simulink model "solar_PV_model"  (R2019a)
settings: Solver=VariableStepAuto  StartTime=0.0  StopTime=80  RelTol=1e-3
undefined symbols (not defined in the file or in its folder): BM, Eg0, Isc, J, K, Kc, ki, La, n, Ns, q, Ra, Rs, Rsh, Tn, Voc
libraries: simulink_extras x4, simulink x2
settings Model: Creator=hermi  LastModifiedBy=hermi

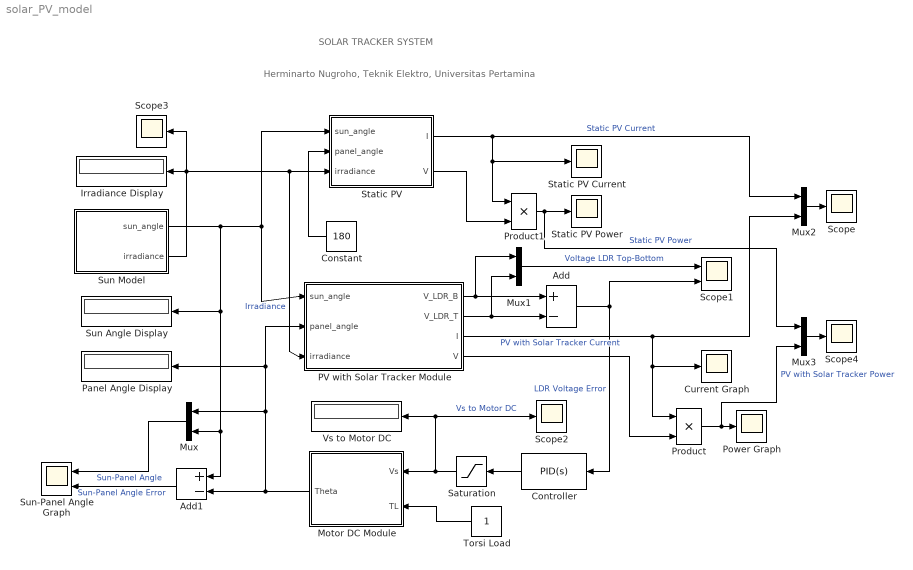
== system solar_PV_model ==
  note: Herminarto Nugroho, Teknik Elektro, Universitas Pertamina
  note: SOLAR TRACKER SYSTEM
  Add : Sum  Inputs=+-
  Add1 : Sum  Inputs=+-
  Constant : Constant  Value=180
  Controller : simulink/Continuous/PID Controller  Controller=PID  Form=Parallel  TimeDomain=Continuous-time  SampleTime=-1  IntegratorMethod=Forward Euler  FilterMethod=Forward Euler  ControllerParametersSource=internal  P=100  I=100  D=0  UseFilter=on  N=100  TunerSelectOption=Transfer Function Based (PID Tuner App)  InitialConditionSource=internal  InitialConditionForIntegrator=0  InitialConditionForFilter=0  DifferentiatorICPrevScaledInput=0  ExternalReset=none  TrackingMode=off  Kt=1  LimitOutput=off  UpperSaturationLimit=180  LowerSaturationLimit=0  LinearizeAsGain=on  AntiWindupMode=none  Kb=1  POutMin=[]  POutMax=[]  IOutMin=[]  IOutMax=[]  DOutMin=[]  DOutMax=[]  NOutMin=[]  NOutMax=[]  SumOutMin=[]  SumOutMax=[]  SaturationOutMin=[]  SaturationOutMax=[]  PParamMin=[]  PParamMax=[]  IParamMin=[]  IParamMax=[]  DParamMin=[]  DParamMax=[]  NParamMin=[]  NParamMax=[]  KbParamMin=[]  KbParamMax=[]  KtParamMin=[]  KtParamMax=[]  KbOutMin=[]  KbOutMax=[]  KtOutMin=[]  KtOutMax=[]  IntegratorOutMin=[]  IntegratorOutMax=[]  FilterOutMin=[]  FilterOutMax=[]  SumI1OutMin=[]  SumI1OutMax=[]  SumI2OutMin=[]  SumI2OutMax=[]  SumI3OutMin=[]  SumI3OutMax=[]  SumI4OutMin=[]  SumI4OutMax=[]  SumDOutMin=[]  SumDOutMax=[]  DifferentiatorOutMin=[]  DifferentiatorOutMax=[]  FilterDiffOutCoefMin=[]  FilterDiffOutCoefMax=[]  ReciprocalOutMin=[]  ReciprocalOutMax=[]  SumDenOutMin=[]  SumDenOutMax=[]  SumNumOutMin=[]  SumNumOutMax=[]  DivideOutMin=[]  DivideOutMax=[]  IntegratorContinuousStateAttributes=''  IntegratorStateMustResolveToSignalObject=off  IntegratorRTWStateStorageClass=Auto  FilterContinuousStateAttributes=''  FilterStateMustResolveToSignalObject=off  FilterRTWStateStorageClass=Auto  ParallelPVariant=InternalParameters  IdealPVariant=Disabled  IVariant=InternalParameters  DVariant=InternalParameters  IntegratorVariant=Continuous  SatVariant=Disabled  AWVariant=Passthrough  PCopyVariant=Disabled  TRVariant=Disabled  FdbkBlocksVariant=Forward  IdealPFdbkVariant=Disabled  SatFdbkVariant=Disabled  DerivativeFilterVariant=ContFilter  NVariant=InternalParameters  NCopyVariant=Disabled  FilterICVariant=InternalICsFilter  IntegratorICVariant=InternalICs  ExternalResetVariant=Disabled  TRSumVariant=Passthrough  SumFdbkVariant=Disabled  SumVariant=Sum_PID
  Current Graph : Scope
  Irradiance Display : Display
  Motor DC Module : Subsystem  InitFcn=|
      | Ra=0.5,
      | La=1.5e-3,
      | Kc=0.05,
      | J=2.5e-4,
      | BM=1e-4,
  Mux{,1..3} (4 alike) : Mux  Inputs=2
  PV with Solar Tracker Module : Subsystem
  Panel Angle Display : Display
  Power Graph : Scope
  Product : Product
  Product1 : Product
  Saturation : Saturate  UpperLimit=12  LowerLimit=-12
  Scope{,2..4} (4 alike) : Scope
  Scope1 : Scope  NumInputPorts=2
  Static PV : Subsystem
  Static PV Current : Scope
  Static PV Power : Scope
  Sun Angle Display : Display
  Sun Model : Subsystem
  Sun-Panel Angle Graph : Scope  NumInputPorts=2
  Torsi Load : Constant
  Vs to Motor DC : Display
  wires:
  PV with Solar Tracker Module/3(I) -> Mux2/2, Current Graph/1, Product/1  "PV with Solar Tracker Current"
  PV with Solar Tracker Module/4(V) -> Product/2
  Product/1 -> Mux3/2, Power Graph/1  "PV with Solar Tracker Power"
  Sun Model/2(irradiance) -> PV with Solar Tracker Module/3(irradiance), Static PV/3(irradiance), Scope3/1, Irradiance Display/1  "Irradiance"
  Motor DC Module/1(Theta) -> Add1/2, Mux/1, Panel Angle Display/1, PV with Solar Tracker Module/2(panel_angle)
  Add/1 -> Scope1/2, Controller/1  "LDR Voltage Error"
  Sun Model/1(sun_angle) -> Add1/1, Mux/2, Sun Angle Display/1, Static PV/1(sun_angle), PV with Solar Tracker Module/1(sun_angle)
  PV with Solar Tracker Module/1(V_LDR_B) -> Mux1/1, Add/1
  PV with Solar Tracker Module/2(V_LDR_T) -> Mux1/2, Add/2
  Torsi Load/1 -> Motor DC Module/2(TL)
  Controller/1 -> Saturation/1
  Saturation/1 -> Scope2/1, Vs to Motor DC/1, Motor DC Module/1(Vs)  "Vs to Motor DC"
  Mux/1 -> Sun-Panel Angle Graph/1  "Sun-Panel Angle"
  Add1/1 -> Sun-Panel Angle Graph/2  "Sun-Panel Angle Error"
  Mux1/1 -> Scope1/1  "Voltage LDR Top-Bottom"
  Product1/1 -> Static PV Power/1, Mux3/1  "Static PV Power"
  Static PV/1(I) -> Product1/1, Static PV Current/1, Mux2/1  "Static PV Current"
  Static PV/2(V) -> Product1/2
  Mux2/1 -> Scope/1
  Constant/1 -> Static PV/2(panel_angle)
  Mux3/1 -> Scope4/1

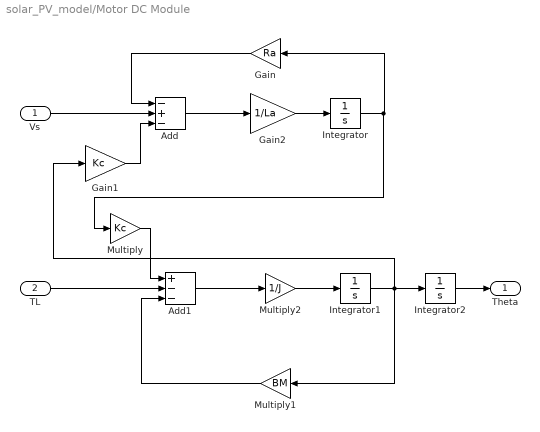
== system solar_PV_model/Motor DC Module ==
  Vs : Inport
  TL : Inport  Port=2
  Add : Sum  Inputs=-+-
  Add1 : Sum  Inputs=+--
  Gain : Gain  Gain=Ra
  Gain1 : Gain  Gain=Kc
  Gain2 : Gain  Gain=1/La
  Integrator : Integrator
  Integrator1 : Integrator
  Integrator2 : Integrator
  Multiply : Gain  Gain=Kc
  Multiply1 : Gain  Gain=BM
  Multiply2 : Gain  Gain=1/J
  Theta : Outport
  wires:
  Gain1/1 -> Add/3
  Gain/1 -> Add/1
  Multiply/1 -> Add1/1
  Add1/1 -> Multiply2/1
  Gain2/1 -> Integrator/1
  TL/1 -> Add1/2
  Multiply2/1 -> Integrator1/1
  Integrator1/1 -> Integrator2/1, Multiply1/1, Gain1/1
  Add/1 -> Gain2/1
  Vs/1 -> Add/2
  Integrator/1 -> Multiply/1, Gain/1
  Multiply1/1 -> Add1/3
  Integrator2/1 -> Theta/1

== system solar_PV_model/PV with Solar Tracker Module ==
  sun_angle : Inport
  panel_angle : Inport  Port=2
  irradiance : Inport  Port=3
  Effective Irradiance Model : Subsystem
  LDR Sensor Module : Subsystem
  PV Module : Subsystem  InitFcn=|
      | ki=0.0032,
      | q=1.6e-19,
      | K=1.38e-23,
      | n=1.3,
      | Eg0=1.1,
      | Rs=0.221,
      | Rsh=414.405,
      | Tn=298,
      | Voc=32.9,
      | Isc=8.21,
      | Ns=54,
  Temperature (C) : Constant  Value=30
  V_LDR_B : Outport
  V_LDR_T : Outport  Port=2
  I : Outport  Port=3
  V : Outport  Port=4
  wires:
  sun_angle/1 -> Effective Irradiance Model/1(sun_angle), LDR Sensor Module/1(sun_angle)
  panel_angle/1 -> Effective Irradiance Model/2(panel_angle), LDR Sensor Module/2(panel_angle)
  Temperature (C)/1 -> PV Module/1(T)
  Effective Irradiance Model/1(effective_irradiance) -> PV Module/2(G)
  LDR Sensor Module/1(V_LDR_B1) -> V_LDR_B/1
  irradiance/1 -> Effective Irradiance Model/3(irradiance), LDR Sensor Module/3(irradiance)
  LDR Sensor Module/2(V_LDR_T1) -> V_LDR_T/1
  PV Module/1(I) -> I/1  "PV Current"
  PV Module/2(V) -> V/1  "V"

== system solar_PV_model/Static PV ==
  sun_angle : Inport
  panel_angle : Inport  Port=2
  irradiance : Inport  Port=3
  Effective Irradiance Model : Subsystem
  PV Module : Subsystem  InitFcn=|
      | ki=0.0032,
      | q=1.6e-19,
      | K=1.38e-23,
      | n=1.3,
      | Eg0=1.1,
      | Rs=0.221,
      | Rsh=414.405,
      | Tn=298,
      | Voc=32.9,
      | Isc=8.21,
      | Ns=54,
  Temperature (C) : Constant  Value=30
  I : Outport
  V : Outport  Port=2
  wires:
  Temperature (C)/1 -> PV Module/1(T)
  Effective Irradiance Model/1(effective_irradiance) -> PV Module/2(G)
  sun_angle/1 -> Effective Irradiance Model/1(sun_angle)
  panel_angle/1 -> Effective Irradiance Model/2(panel_angle)
  irradiance/1 -> Effective Irradiance Model/3(irradiance)
  PV Module/1(I) -> I/1  "PV Current"
  PV Module/2(V) -> V/1  "V"

== system solar_PV_model/Sun Model ==
  15_deg/hr : Constant  Value=15/60
  MATLAB Function : MATLAB Function  TreatAsAtomicUnit=on
  Product1 : Product
  Saturation : Saturate  UpperLimit=18*60  LowerLimit=6*60
  Starting 6 am : simulink/Sources/Ramp  slope=10  start=0  InitialOutput=6*60
  sun_angle : Outport
  irradiance : Outport  Port=2
  wires:
  15_deg/hr/1 -> Product1/2
  Starting 6 am/1 -> Saturation/1
  MATLAB Function/1(X) -> irradiance/1
  Saturation/1 -> MATLAB Function/1(x), Product1/1
  Product1/1 -> sun_angle/1

== system solar_PV_model/PV with Solar Tracker Module/Effective Irradiance Model ==
  sun_angle : Inport
  panel_angle : Inport  Port=2
  irradiance : Inport  Port=3
  Add : Sum  Inputs=+-
  Cos : Trigonometry  Operator=cos
  Degrees to Radians : simulink_extras/Transformations/Degrees to Radians
  Product2 : Product  Inputs=**
  Saturation : Saturate  UpperLimit=90  LowerLimit=-90
  effective_irradiance : Outport
  wires:
  sun_angle/1 -> Add/1
  Cos/1 -> Product2/1
  Product2/1 -> effective_irradiance/1
  Degrees to Radians/1 -> Cos/1
  Add/1 -> Degrees to Radians/1
  panel_angle/1 -> Add/2
  irradiance/1 -> Product2/2

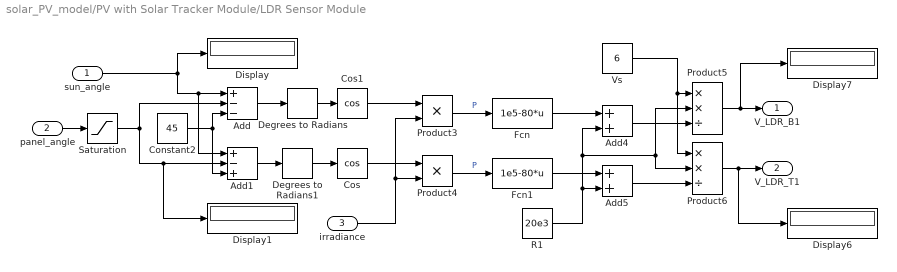
== system solar_PV_model/PV with Solar Tracker Module/LDR Sensor Module ==
  sun_angle : Inport
  panel_angle : Inport  Port=2
  irradiance : Inport  Port=3
  Add : Sum  Inputs=+--
  Add1 : Sum  Inputs=+-+
  Add4 : Sum
  Add5 : Sum
  Constant2 : Constant  Value=45
  Cos : Trigonometry  Operator=cos
  Cos1 : Trigonometry  Operator=cos
  Degrees to Radians : simulink_extras/Transformations/Degrees to Radians
  Degrees to Radians1 : simulink_extras/Transformations/Degrees to Radians
  Display{,1,6..7} (4 alike) : Display
  Fcn : Fcn  Expr=1e5-80*u
  Fcn1 : Fcn  Expr=1e5-80*u
  Product3 : Product
  Product4 : Product
  Product5 : Product  Inputs=**/
  Product6 : Product  Inputs=**/
  R1 : Constant  Value=20e3
  Saturation : Saturate  UpperLimit=360  LowerLimit=0
  Vs : Constant  Value=6
  V_LDR_B1 : Outport
  V_LDR_T1 : Outport  Port=2
  wires:
  Product6/1 -> Display6/1, V_LDR_T1/1
  Add4/1 -> Product5/3
  Vs/1 -> Product6/1, Product5/1
  R1/1 -> Add5/2, Product6/2, Product5/2, Add4/2
  irradiance/1 -> Product4/2, Product3/2
  Degrees to Radians1/1 -> Cos/1
  Add5/1 -> Product6/3
  Product5/1 -> Display7/1, V_LDR_B1/1
  Add1/1 -> Degrees to Radians1/1
  Cos1/1 -> Product3/1
  Product4/1 -> Fcn1/1  "P"
  Cos/1 -> Product4/1
  Fcn/1 -> Add4/1
  Product3/1 -> Fcn/1  "P"
  Add/1 -> Degrees to Radians/1
  Constant2/1 -> Add1/3, Add/3
  Degrees to Radians/1 -> Cos1/1
  panel_angle/1 -> Saturation/1
  sun_angle/1 -> Add1/1, Add/1, Display/1
  Fcn1/1 -> Add5/1
  Saturation/1 -> Add/2, Display1/1, Add1/2

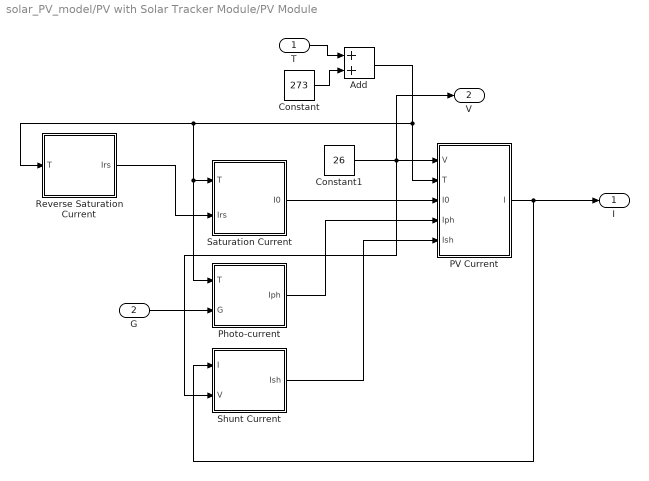
== system solar_PV_model/PV with Solar Tracker Module/PV Module ==
  T : Inport
  G : Inport  Port=2
  Add : Sum
  Constant : Constant  Value=273
  Constant1 : Constant  Value=26
  PV Current : Subsystem
  Photo-current : Subsystem
  Reverse Saturation Current : Subsystem
  Saturation Current : Subsystem
  Shunt Current : Subsystem
  I : Outport
  V : Outport  Port=2
  wires:
  Photo-current/1(Iph) -> PV Current/4(Iph)
  Saturation Current/1(I0) -> PV Current/3(I0)
  PV Current/1(I) -> I/1, Shunt Current/1(I)
  G/1 -> Photo-current/2(G)
  Add/1 -> PV Current/2(T), Reverse Saturation Current/1(T), Saturation Current/1(T), Photo-current/1(T)
  Constant/1 -> Add/2
  Constant1/1 -> V/1, Shunt Current/2(V), PV Current/1(V)
  Shunt Current/1(Ish) -> PV Current/5(Ish)
  Reverse Saturation Current/1(Irs) -> Saturation Current/2(Irs)
  T/1 -> Add/1

== system solar_PV_model/Static PV/Effective Irradiance Model ==
  sun_angle : Inport
  panel_angle : Inport  Port=2
  irradiance : Inport  Port=3
  Add : Sum  Inputs=+-
  Cos : Trigonometry  Operator=cos
  Degrees to Radians : simulink_extras/Transformations/Degrees to Radians
  Product2 : Product  Inputs=**
  Saturation : Saturate  UpperLimit=90  LowerLimit=-90
  effective_irradiance : Outport
  wires:
  sun_angle/1 -> Add/1
  Cos/1 -> Product2/1
  Product2/1 -> effective_irradiance/1
  Degrees to Radians/1 -> Cos/1
  Add/1 -> Degrees to Radians/1
  panel_angle/1 -> Add/2
  irradiance/1 -> Product2/2

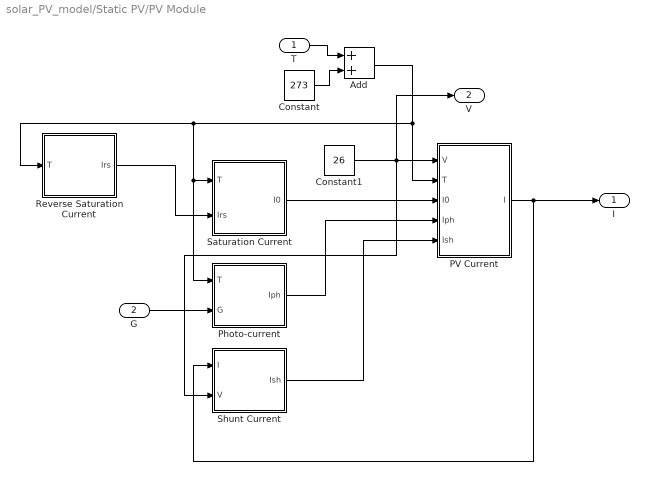
== system solar_PV_model/Static PV/PV Module ==
  T : Inport
  G : Inport  Port=2
  Add : Sum
  Constant : Constant  Value=273
  Constant1 : Constant  Value=26
  PV Current : Subsystem
  Photo-current : Subsystem
  Reverse Saturation Current : Subsystem
  Saturation Current : Subsystem
  Shunt Current : Subsystem
  I : Outport
  V : Outport  Port=2
  wires:
  Photo-current/1(Iph) -> PV Current/4(Iph)
  Saturation Current/1(I0) -> PV Current/3(I0)
  PV Current/1(I) -> I/1, Shunt Current/1(I)
  G/1 -> Photo-current/2(G)
  Add/1 -> PV Current/2(T), Reverse Saturation Current/1(T), Saturation Current/1(T), Photo-current/1(T)
  Constant/1 -> Add/2
  Constant1/1 -> V/1, Shunt Current/2(V), PV Current/1(V)
  Shunt Current/1(Ish) -> PV Current/5(Ish)
  Reverse Saturation Current/1(Irs) -> Saturation Current/2(Irs)
  T/1 -> Add/1

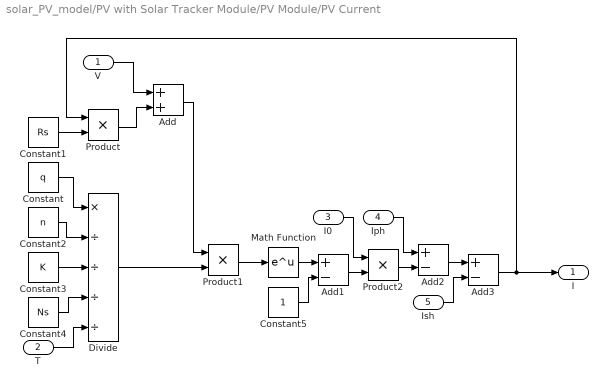
== system solar_PV_model/PV with Solar Tracker Module/PV Module/PV Current ==
  V : Inport
  T : Inport  Port=2
  I0 : Inport  Port=3
  Iph : Inport  Port=4
  Ish : Inport  Port=5
  Add : Sum
  Add1 : Sum  Inputs=+-
  Add2 : Sum  Inputs=+-
  Add3 : Sum  Inputs=+-
  Constant : Constant  Value=q
  Constant1 : Constant  Value=Rs
  Constant2 : Constant  Value=n
  Constant3 : Constant  Value=K
  Constant4 : Constant  Value=Ns
  Constant5 : Constant
  Divide : Product  Inputs=*////
  Math Function : Math  SaturateOnIntegerOverflow=on
  Product : Product
  Product1 : Product
  Product2 : Product
  I : Outport
  wires:
  Constant5/1 -> Add1/2
  Add1/1 -> Product2/2
  Constant3/1 -> Divide/3
  Add/1 -> Product1/1
  T/1 -> Divide/5
  Divide/1 -> Product1/2
  Constant2/1 -> Divide/2
  Product1/1 -> Math Function/1
  Product2/1 -> Add2/2
  Iph/1 -> Add2/1
  Math Function/1 -> Add1/1
  Constant1/1 -> Product/2
  Product/1 -> Add/2
  V/1 -> Add/1
  I0/1 -> Product2/1
  Constant/1 -> Divide/1
  Add2/1 -> Add3/1
  Add3/1 -> I/1, Product/1
  Constant4/1 -> Divide/4
  Ish/1 -> Add3/2

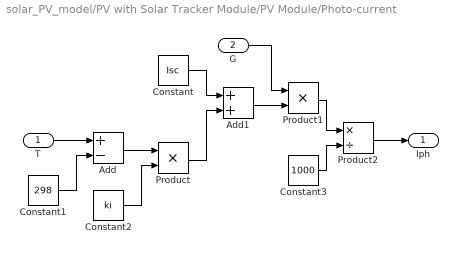
== system solar_PV_model/PV with Solar Tracker Module/PV Module/Photo-current ==
  T : Inport
  G : Inport  Port=2
  Add : Sum  Inputs=+-
  Add1 : Sum
  Constant : Constant  Value=Isc
  Constant1 : Constant  Value=298
  Constant2 : Constant  Value=ki
  Constant3 : Constant  Value=1000
  Product : Product
  Product1 : Product
  Product2 : Product  Inputs=*/
  Iph : Outport
  wires:
  T/1 -> Add/1
  Add/1 -> Product/1
  Constant/1 -> Add1/1
  Product1/1 -> Product2/1
  Product2/1 -> Iph/1
  G/1 -> Product1/1
  Add1/1 -> Product1/2
  Constant3/1 -> Product2/2
  Constant1/1 -> Add/2
  Constant2/1 -> Product/2
  Product/1 -> Add1/2

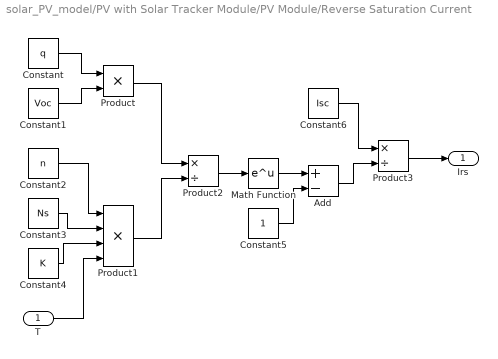
== system solar_PV_model/PV with Solar Tracker Module/PV Module/Reverse Saturation Current ==
  T : Inport
  Add : Sum  Inputs=+-
  Constant : Constant  Value=q
  Constant1 : Constant  Value=Voc
  Constant2 : Constant  Value=n
  Constant3 : Constant  Value=Ns
  Constant4 : Constant  Value=K
  Constant5 : Constant
  Constant6 : Constant  Value=Isc
  Math Function : Math  SaturateOnIntegerOverflow=on
  Product : Product
  Product1 : Product  Inputs=****
  Product2 : Product  Inputs=*/
  Product3 : Product  Inputs=*/
  Irs : Outport
  wires:
  Add/1 -> Product3/2
  Constant3/1 -> Product1/2
  Product1/1 -> Product2/2
  Constant6/1 -> Product3/1
  Constant5/1 -> Add/2
  Constant4/1 -> Product1/3
  Constant1/1 -> Product/2
  Product3/1 -> Irs/1
  Math Function/1 -> Add/1
  Product/1 -> Product2/1
  Constant2/1 -> Product1/1
  Product2/1 -> Math Function/1
  Constant/1 -> Product/1
  T/1 -> Product1/4

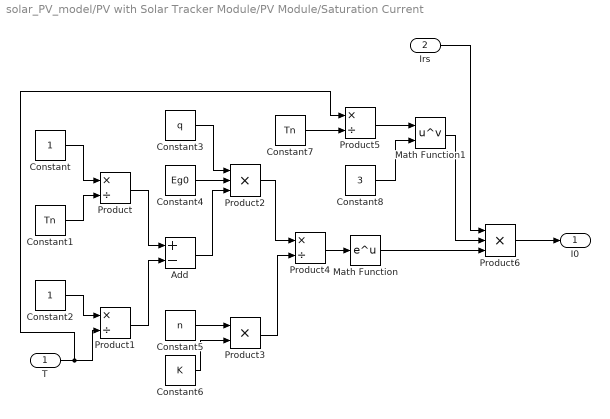
== system solar_PV_model/PV with Solar Tracker Module/PV Module/Saturation Current ==
  T : Inport
  Irs : Inport  Port=2
  Add : Sum  Inputs=+-
  Constant : Constant
  Constant1 : Constant  Value=Tn
  Constant2 : Constant
  Constant3 : Constant  Value=q
  Constant4 : Constant  Value=Eg0
  Constant5 : Constant  Value=n
  Constant6 : Constant  Value=K
  Constant7 : Constant  Value=Tn
  Constant8 : Constant  Value=3
  Math Function : Math  SaturateOnIntegerOverflow=on
  Math Function1 : Math  Operator=pow  SaturateOnIntegerOverflow=on
  Product{,1,4..5} (4 alike) : Product  Inputs=*/
  Product2 : Product  Inputs=***
  Product3 : Product  Inputs=**
  Product6 : Product  Inputs=***
  I0 : Outport
  wires:
  Constant6/1 -> Product3/2
  Math Function1/1 -> Product6/2
  Constant4/1 -> Product2/2
  T/1 -> Product1/2, Product5/1
  Constant5/1 -> Product3/1
  Constant3/1 -> Product2/1
  Constant8/1 -> Math Function1/2
  Product1/1 -> Add/2
  Constant7/1 -> Product5/2
  Add/1 -> Product2/3
  Product4/1 -> Math Function/1
  Math Function/1 -> Product6/3
  Irs/1 -> Product6/1
  Product5/1 -> Math Function1/1
  Product2/1 -> Product4/1
  Product3/1 -> Product4/2
  Constant/1 -> Product/1
  Constant1/1 -> Product/2
  Constant2/1 -> Product1/1
  Product6/1 -> I0/1
  Product/1 -> Add/1

== system solar_PV_model/PV with Solar Tracker Module/PV Module/Shunt Current ==
  I : Inport
  V : Inport  Port=2
  Add : Sum
  Constant : Constant  Value=Rs
  Constant1 : Constant  Value=Rsh
  Product : Product
  Product1 : Product  Inputs=*/
  Ish : Outport
  wires:
  Product1/1 -> Ish/1
  I/1 -> Product/1
  V/1 -> Add/2
  Add/1 -> Product1/1
  Product/1 -> Add/1
  Constant/1 -> Product/2
  Constant1/1 -> Product1/2

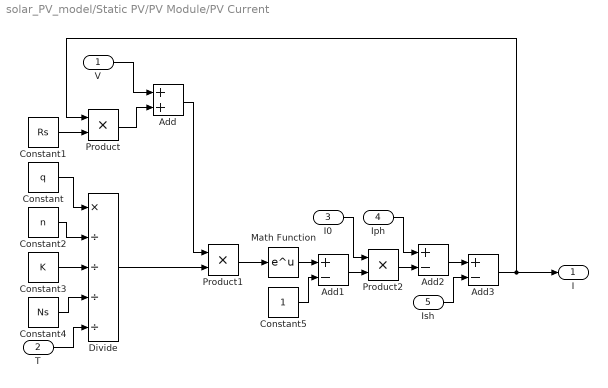
== system solar_PV_model/Static PV/PV Module/PV Current ==
  V : Inport
  T : Inport  Port=2
  I0 : Inport  Port=3
  Iph : Inport  Port=4
  Ish : Inport  Port=5
  Add : Sum
  Add1 : Sum  Inputs=+-
  Add2 : Sum  Inputs=+-
  Add3 : Sum  Inputs=+-
  Constant : Constant  Value=q
  Constant1 : Constant  Value=Rs
  Constant2 : Constant  Value=n
  Constant3 : Constant  Value=K
  Constant4 : Constant  Value=Ns
  Constant5 : Constant
  Divide : Product  Inputs=*////
  Math Function : Math  SaturateOnIntegerOverflow=on
  Product : Product
  Product1 : Product
  Product2 : Product
  I : Outport
  wires:
  Constant5/1 -> Add1/2
  Add1/1 -> Product2/2
  Constant3/1 -> Divide/3
  Add/1 -> Product1/1
  T/1 -> Divide/5
  Divide/1 -> Product1/2
  Constant2/1 -> Divide/2
  Product1/1 -> Math Function/1
  Product2/1 -> Add2/2
  Iph/1 -> Add2/1
  Math Function/1 -> Add1/1
  Constant1/1 -> Product/2
  Product/1 -> Add/2
  V/1 -> Add/1
  I0/1 -> Product2/1
  Constant/1 -> Divide/1
  Add2/1 -> Add3/1
  Add3/1 -> I/1, Product/1
  Constant4/1 -> Divide/4
  Ish/1 -> Add3/2

== system solar_PV_model/Static PV/PV Module/Photo-current ==
  T : Inport
  G : Inport  Port=2
  Add : Sum  Inputs=+-
  Add1 : Sum
  Constant : Constant  Value=Isc
  Constant1 : Constant  Value=298
  Constant2 : Constant  Value=ki
  Constant3 : Constant  Value=1000
  Product : Product
  Product1 : Product
  Product2 : Product  Inputs=*/
  Iph : Outport
  wires:
  T/1 -> Add/1
  Add/1 -> Product/1
  Constant/1 -> Add1/1
  Product1/1 -> Product2/1
  Product2/1 -> Iph/1
  G/1 -> Product1/1
  Add1/1 -> Product1/2
  Constant3/1 -> Product2/2
  Constant1/1 -> Add/2
  Constant2/1 -> Product/2
  Product/1 -> Add1/2

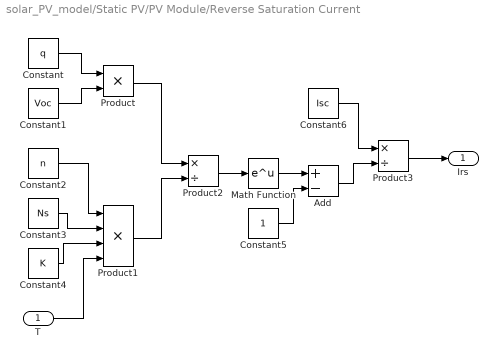
== system solar_PV_model/Static PV/PV Module/Reverse Saturation Current ==
  T : Inport
  Add : Sum  Inputs=+-
  Constant : Constant  Value=q
  Constant1 : Constant  Value=Voc
  Constant2 : Constant  Value=n
  Constant3 : Constant  Value=Ns
  Constant4 : Constant  Value=K
  Constant5 : Constant
  Constant6 : Constant  Value=Isc
  Math Function : Math  SaturateOnIntegerOverflow=on
  Product : Product
  Product1 : Product  Inputs=****
  Product2 : Product  Inputs=*/
  Product3 : Product  Inputs=*/
  Irs : Outport
  wires:
  Add/1 -> Product3/2
  Constant3/1 -> Product1/2
  Product1/1 -> Product2/2
  Constant6/1 -> Product3/1
  Constant5/1 -> Add/2
  Constant4/1 -> Product1/3
  Constant1/1 -> Product/2
  Product3/1 -> Irs/1
  Math Function/1 -> Add/1
  Product/1 -> Product2/1
  Constant2/1 -> Product1/1
  Product2/1 -> Math Function/1
  Constant/1 -> Product/1
  T/1 -> Product1/4

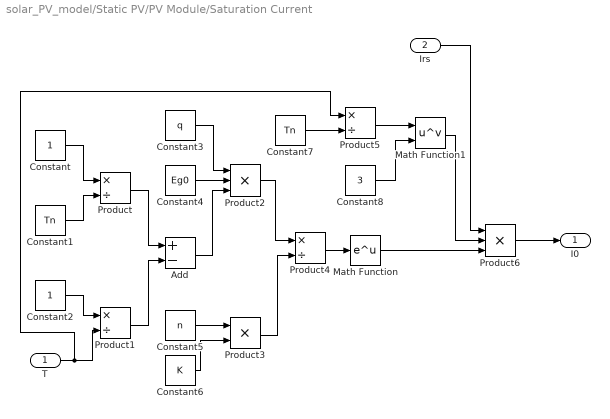
== system solar_PV_model/Static PV/PV Module/Saturation Current ==
  T : Inport
  Irs : Inport  Port=2
  Add : Sum  Inputs=+-
  Constant : Constant
  Constant1 : Constant  Value=Tn
  Constant2 : Constant
  Constant3 : Constant  Value=q
  Constant4 : Constant  Value=Eg0
  Constant5 : Constant  Value=n
  Constant6 : Constant  Value=K
  Constant7 : Constant  Value=Tn
  Constant8 : Constant  Value=3
  Math Function : Math  SaturateOnIntegerOverflow=on
  Math Function1 : Math  Operator=pow  SaturateOnIntegerOverflow=on
  Product{,1,4..5} (4 alike) : Product  Inputs=*/
  Product2 : Product  Inputs=***
  Product3 : Product  Inputs=**
  Product6 : Product  Inputs=***
  I0 : Outport
  wires:
  Constant6/1 -> Product3/2
  Math Function1/1 -> Product6/2
  Constant4/1 -> Product2/2
  T/1 -> Product1/2, Product5/1
  Constant5/1 -> Product3/1
  Constant3/1 -> Product2/1
  Constant8/1 -> Math Function1/2
  Product1/1 -> Add/2
  Constant7/1 -> Product5/2
  Add/1 -> Product2/3
  Product4/1 -> Math Function/1
  Math Function/1 -> Product6/3
  Irs/1 -> Product6/1
  Product5/1 -> Math Function1/1
  Product2/1 -> Product4/1
  Product3/1 -> Product4/2
  Constant/1 -> Product/1
  Constant1/1 -> Product/2
  Constant2/1 -> Product1/1
  Product6/1 -> I0/1
  Product/1 -> Add/1

== system solar_PV_model/Static PV/PV Module/Shunt Current ==
  I : Inport
  V : Inport  Port=2
  Add : Sum
  Constant : Constant  Value=Rs
  Constant1 : Constant  Value=Rsh
  Product : Product
  Product1 : Product  Inputs=*/
  Ish : Outport
  wires:
  Product1/1 -> Ish/1
  I/1 -> Product/1
  V/1 -> Add/2
  Add/1 -> Product1/1
  Product/1 -> Add/1
  Constant/1 -> Product/2
  Constant1/1 -> Product1/2

== matlab function solar_PV_model/Sun Model/MATLAB Function ==
  data: x input; X output
function X = irradiance_m(x)
a0 = 302.1332; a1 = -372.9955; b1 = -250.6906; a2 = 49.4091; b2 = 146.8812; w = 0.005191; 
X =  a0 + a1*cos(x*w) + b1*sin(x*w) + a2*cos(2*x*w) + b2*sin(2*x*w);
